simulink model "sl_subsys_fcncallerr11"  (Simulink 7.6)
settings: Solver=FixedStepDiscrete  StartTime=0.0  StopTime=10.0  FixedStep=1  RelTol=1e-3
undefined symbols (not defined in the file or in its folder): DiscIntNeverNeededParam
Description:
  | Function-call subsystems that incorrectly specify periodic execution
  | 
  | The function-call subsystems below specify a periodic sample time.  This means
  | that their function-call initiators must execute them exactly once per time step.
  | In this example, the function-call initiator is a Stateflow chart that attempts to
  | execute the function-call subsystems twice per time step, or effectively double the
  | specified rate.  As a result Simulink reports an error during simulation.
settings Model: Creator=The MathWorks Inc.  CovMetricSettings=d  ExtModeAutoUpdateStatusClock=off
settings DataIOCC: SignalLoggingName=logsOut
settings OptimizationCC: BlockReduction=off  BooleanDataType=off  InlineInvariantSignals=on  InitFltsAndDblsToZero=on  OptimizeModelRefInitCode=on  LifeSpan=1
settings DebuggingCC: SaveWithParameterizedLinksMsg=none  CheckExecutionContextPreStartOutputMsg=on  CheckExecutionContextRuntimeOutputMsg=on  SignalResolutionControl=TryResolveAllWithWarning  SolverPrmCheckMsg=none  MultiTaskDSMMsg=warning  MultiTaskCondExecSysMsg=none
settings ModelReferenceCC: UpdateModelReferenceTargets=IfOutOfDate
settings SFSimCC: SimParseCustomCode=off
settings RTWCC: SystemTargetFile=ert.tlc  TemplateMakefile=ert_default_tmf  Description=RTW Embedded Coder (no auto configuration)  GenerateReport=on  ProcessScript=ert_make_rtw_hook  IncludeHyperlinkInReport=on  LaunchReport=on  IncludeERTFirstTime=on
settings CodeAppCC: IgnoreCustomStorageClasses=off  CustomSymbolStrFcn=$F$N$M
settings ERTTargetCC: TargetFcnLib=ansi_tfl_tmw.mat  MultiwordLength=2048  GenerateSampleERTMain=on  ERTCustomFileTemplate=example_file_process.tlc  ConvertIfToSwitch=off

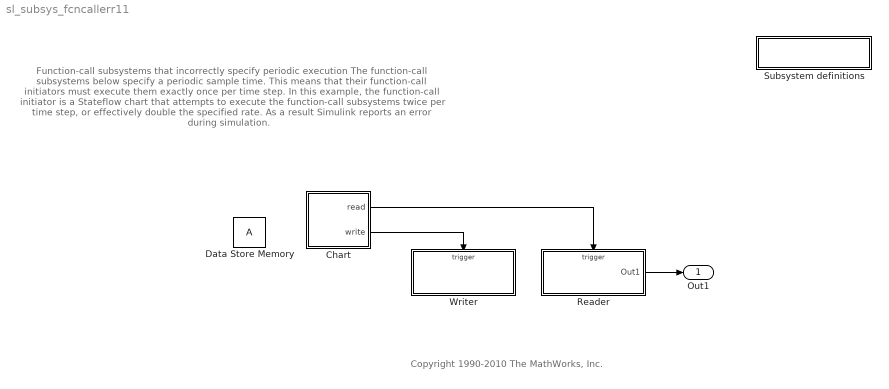
== system sl_subsys_fcncallerr11 ==
  note: Function-call subsystems that incorrectly specify periodic execution
      |
      | The function-call subsystems below specify a periodic sample time.  This means
      | that their function-call initiators must execute them exactly once per time step.
      | In this example, the function-call initiator is a Stateflow chart that attempts to
      | execute the function-call subsystems twice per time step, or effectively double the
      | specified rate.  As a result Simulink reports an error during simulation.
  note: Copyright 1990-2010 The MathWorks, Inc.
  " Subsystem definitions" : Subsystem
      settings: OpenFcn=helpview([matlabroot,'/toolbox/simulink/simdemos/simfeatures/html/sl_subsys_definitions.html']);
      mask Display: disp('Subsystem\ndefinitions')
  Chart : Stateflow chart  TreatAsAtomicUnit=on
  Data Store Memory : DataStoreMemory
  Reader : Subsystem  TreatAsAtomicUnit=on
  Writer : Subsystem  TreatAsAtomicUnit=on
  Out1 : Outport
  wires:
  Reader/1(Out1) -> Out1/1
  Chart/1(read) -> Reader/Trigger
  Chart/2(write) -> Writer/Trigger

== system sl_subsys_fcncallerr11/ Subsystem definitions ==

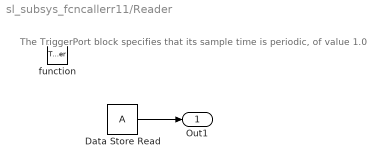
== system sl_subsys_fcncallerr11/Reader ==
  note: The TriggerPort block specifies that its
      | sample time is periodic, of value 1.0
  function : TriggerPort  TriggerType=function-call  SampleTimeType=periodic
  Data Store Read : DataStoreRead
  Out1 : Outport
  wires:
  Data Store Read/1 -> Out1/1

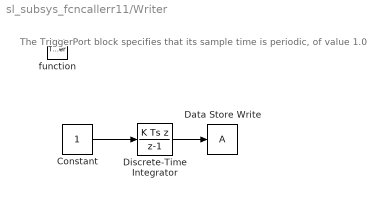
== system sl_subsys_fcncallerr11/Writer ==
  note: The TriggerPort block specifies that its
      | sample time is periodic, of value 1.0
  function : TriggerPort  TriggerType=function-call  SampleTimeType=periodic
  Constant : Constant
  Data Store Write : DataStoreWrite
  Discrete-Time Integrator : DiscreteIntegrator  IntegratorMethod=Integration: Backward Euler  SampleTime=-1  ICPrevOutput=DiscIntNeverNeededParam  ICPrevScaledInput=DiscIntNeverNeededParam
  wires:
  Constant/1 -> Discrete-Time Integrator/1
  Discrete-Time Integrator/1 -> Data Store Write/1

== stateflow chart Chart ==
  (default) -> (junction 3) : {write; read; write; read;}
  events: read output FUNCTION_CALL_EVENT; write output FUNCTION_CALL_EVENT
